simulink model "board_parameters"  (R2020b)
settings: Solver=FixedStepAuto  StartTime=0.0  StopTime=10.0  FixedStep=1e-3  RelTol=1e-3  EnableMultiTasking=on
undefined symbols (not defined in the file): D10, D11, D12, D13, D2, D3, D4, D5, D6, D7, D8, D9, PTA0, PTA1, PTA2, PTB23, PTB9, PTC2, PTC3, PTC4, PTD0, PTD1, PTD2, PTD3
libraries: frdmk64flib x12
settings Model: ExtModeTrigDuration=5  Creator=Sebastian  LastModifiedBy=Sebastian
settings OptimizationCC: EnhancedBackFolding=on  PassReuseOutputArgsAs=Individual arguments  ZeroExternalMemoryAtStartup=off  ZeroInternalMemoryAtStartup=off  MaxStackSize=64  OptimizeBlockOrder=speed  DifferentSizesBufferReuse=on  OptimizationCustomize=off  EfficientTunableParamExpr=on
settings DebuggingCC: ParameterTunabilityLossMsg=error
settings HardwareCC: ProdBitPerPointer=32  ProdBitPerSizeT=32  ProdBitPerPtrDiffT=32  ProdLargestAtomicInteger=Long  ProdLargestAtomicFloat=Double  ProdWordSize=32  ProdHWDeviceType=ARM Compatible->ARM Cortex
settings SFSimCC: MATLABDynamicMemAlloc=off
settings RTWCC: Description=Embedded Coder  SystemTargetFile=ert.tlc  HardwareBoard=NXP FRDM-K64F  TLCOptions="-aInlineSetEventsForThisBaseRateFcn=TLC_FALSE -aSuppressMultiTaskScheduler=TLC_FALSE  -aRateBasedStepFcn=0"  TemplateMakefile=ert_default_tmf  Toolchain=GNU Tools for ARM Embedded Processors
settings CodeAppCC: ForceParamTrailComments=on  IgnoreCustomStorageClasses=off  OperatorAnnotations=on  SimulinkDataObjDesc=on  SFDataObjDesc=on  InsertBlockDesc=on
settings ERTTargetCC: ExtModeTransport=4  ExtModeMexFile=sendToCommService

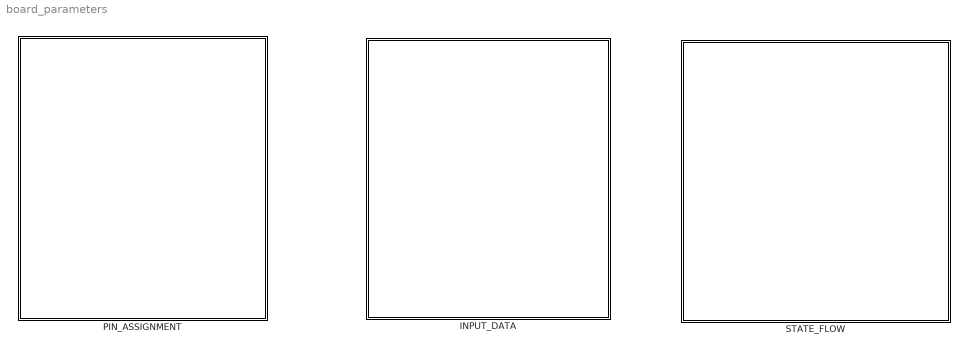
== system board_parameters ==
  INPUT_DATA : Subsystem
  PIN_ASSIGNMENT : Subsystem
  STATE_FLOW : Subsystem

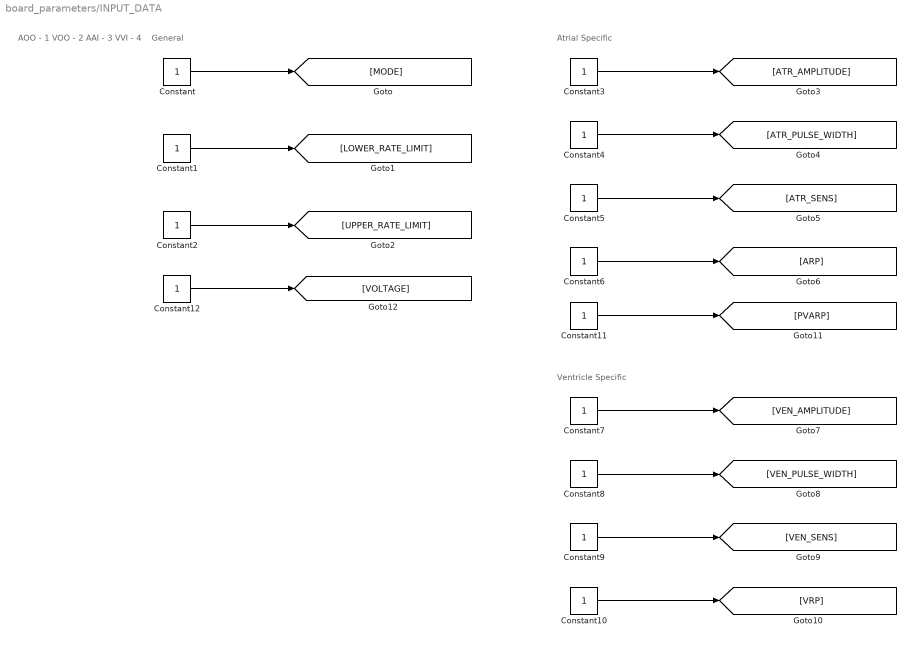
== system board_parameters/INPUT_DATA ==
  note: Atrial Specific
  note: General
  note: AOO - 1
      | VOO - 2
      | AAI - 3
      | VVI - 4
  note: Ventricle Specific
  Constant{,1..12} (13 alike) : Constant
  wires:
  Constant/1 -> [MODE]
  Constant1/1 -> [LOWER_RATE_LIMIT]
  Constant2/1 -> [UPPER_RATE_LIMIT]
  Constant3/1 -> [ATR_AMPLITUDE]
  Constant4/1 -> [ATR_PULSE_WIDTH]
  Constant5/1 -> [ATR_SENS]
  Constant6/1 -> [ARP]
  Constant10/1 -> [VRP]
  Constant9/1 -> [VEN_SENS]
  Constant8/1 -> [VEN_PULSE_WIDTH]
  Constant7/1 -> [VEN_AMPLITUDE]
  Constant11/1 -> [PVARP]
  Constant12/1 -> [VOLTAGE]

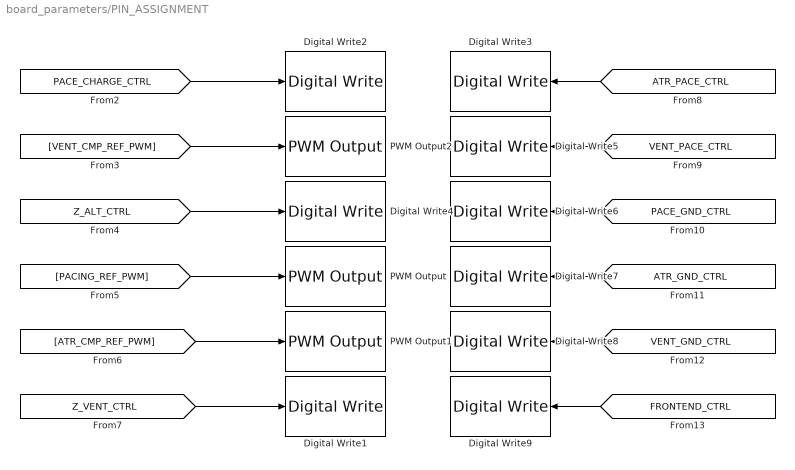
== system board_parameters/PIN_ASSIGNMENT ==
  Digital Write1 : frdmk64flib/Digital Write  Whichpin=PTC3 (D7)
  Digital Write2 : frdmk64flib/Digital Write  Whichpin=PTB9 (D2)
  Digital Write3 : frdmk64flib/Digital Write  Whichpin=PTA0 (D8)
  Digital Write4 : frdmk64flib/Digital Write  Whichpin=PTB23 (D4)
  Digital Write5 : frdmk64flib/Digital Write  Whichpin=PTC4 (D9)
  Digital Write6 : frdmk64flib/Digital Write  Whichpin=PTD0 (D10)
  Digital Write7 : frdmk64flib/Digital Write  Whichpin=PTD2 (D11)
  Digital Write8 : frdmk64flib/Digital Write  Whichpin=PTD3 (D12)
  Digital Write9 : frdmk64flib/Digital Write  Whichpin=PTD1 (D13)
  PWM Output : frdmk64flib/PWM Output  Whichpin=PTA2 (D5)  InitialFrequency=2000  InitialDutyCycle=0
  PWM Output1 : frdmk64flib/PWM Output  Whichpin=PTC2 (D6)  InitialFrequency=2000  InitialDutyCycle=0
  PWM Output2 : frdmk64flib/PWM Output  Whichpin=PTA1 (D3)  InitialFrequency=2000  InitialDutyCycle=0
  wires:
  [ATR_CMP_REF_PWM] -> PWM Output1/1
  [VENT_CMP_REF_PWM] -> PWM Output2/1
  [VENT_PACE_CTRL] -> Digital Write5/1
  [PACE_GND_CTRL] -> Digital Write6/1
  [PACING_REF_PWM] -> PWM Output/1
  [ATR_PACE_CTRL] -> Digital Write3/1
  [FRONTEND_CTRL] -> Digital Write9/1
  [ATR_GND_CTRL] -> Digital Write7/1
  [VENT_GND_CTRL] -> Digital Write8/1
  [PACE_CHARGE_CTRL] -> Digital Write2/1
  [Z_VENT_CTRL] -> Digital Write1/1
  [Z_ALT_CTRL] -> Digital Write4/1

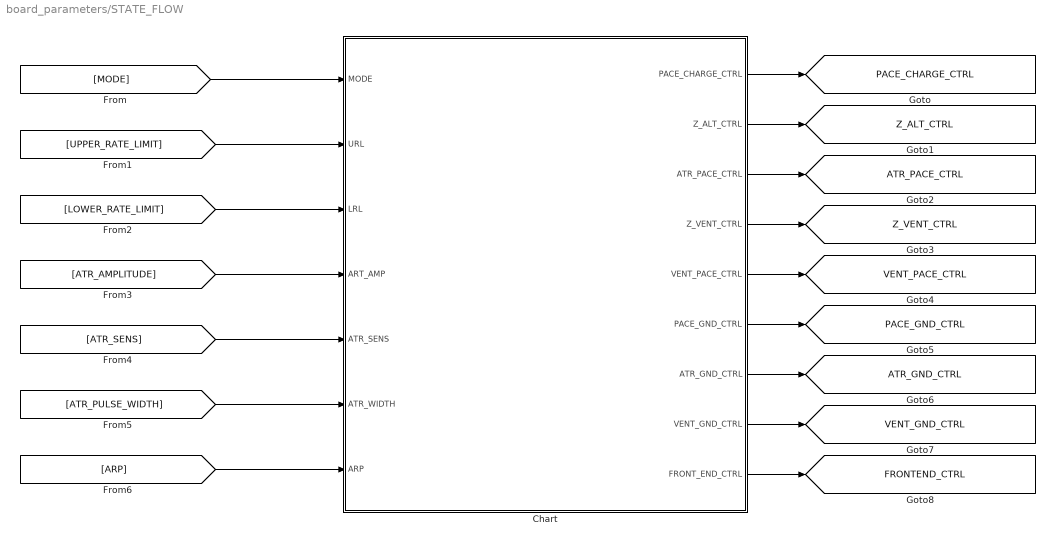
== system board_parameters/STATE_FLOW ==
  Chart : Stateflow chart  TreatAsAtomicUnit=on
  tag scope: ATR_GND_CTRL=global, ATR_PACE_CTRL=global, FRONTEND_CTRL=global, PACE_CHARGE_CTRL=global, PACE_GND_CTRL=global, VENT_GND_CTRL=global, VENT_PACE_CTRL=global, Z_ALT_CTRL=global, Z_VENT_CTRL=global
  wires:
  Chart/1(PACE_CHARGE_CTRL) -> [PACE_CHARGE_CTRL]
  Chart/2(Z_ALT_CTRL) -> [Z_ALT_CTRL]
  Chart/3(ATR_PACE_CTRL) -> [ATR_PACE_CTRL]
  Chart/4(Z_VENT_CTRL) -> [Z_VENT_CTRL]
  Chart/5(VENT_PACE_CTRL) -> [VENT_PACE_CTRL]
  Chart/6(PACE_GND_CTRL) -> [PACE_GND_CTRL]
  Chart/7(ATR_GND_CTRL) -> [ATR_GND_CTRL]
  Chart/8(VENT_GND_CTRL) -> [VENT_GND_CTRL]
  Chart/9(FRONT_END_CTRL) -> [FRONTEND_CTRL]
  [MODE] -> Chart/1(MODE)
  [UPPER_RATE_LIMIT] -> Chart/2(URL)
  [LOWER_RATE_LIMIT] -> Chart/3(LRL)
  [ATR_AMPLITUDE] -> Chart/4(ART_AMP)
  [ATR_SENS] -> Chart/5(ATR_SENS)
  [ATR_PULSE_WIDTH] -> Chart/6(ATR_WIDTH)
  [ARP] -> Chart/7(ARP)

== stateflow chart board_parameters/STATE_FLOW/Chart ==
  data: MODE input; URL input; LRL input; ART_AMP input; ATR_SENS input; ATR_WIDTH input; ARP input; PACE_CHARGE_CTRL output; Z_ALT_CTRL output; ATR_PACE_CTRL output; Z_VENT_CTRL output; VENT_PACE_CTRL output; PACE_GND_CTRL output; ATR_GND_CTRL output; VENT_GND_CTRL output; FRONT_END_CTRL output
